simulink subsystem "Compute_Environments"  (R2025b)
settings: Solver=VariableStepAuto  StartTime=0.0  StopTime=10.0  RelTol=1e-3
undefined symbols (not defined in the file): alpha_temp, Cbar, g0, gamma, h_0_2, magnitude, mu0, P_0_1, P_0_2, r_planet_radius, Rair, rho_0_1, rho_0_2, S, T_0_1, T_0_2
settings Model: Creator=Kat  LastModifiedBy=cdriggs

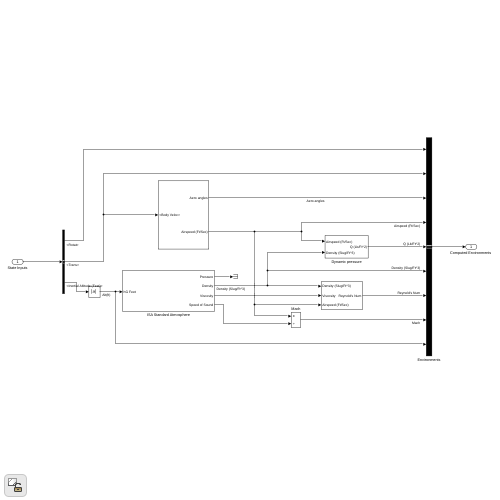
[thumbnail: Simulink's stored preview of the top-level diagram]
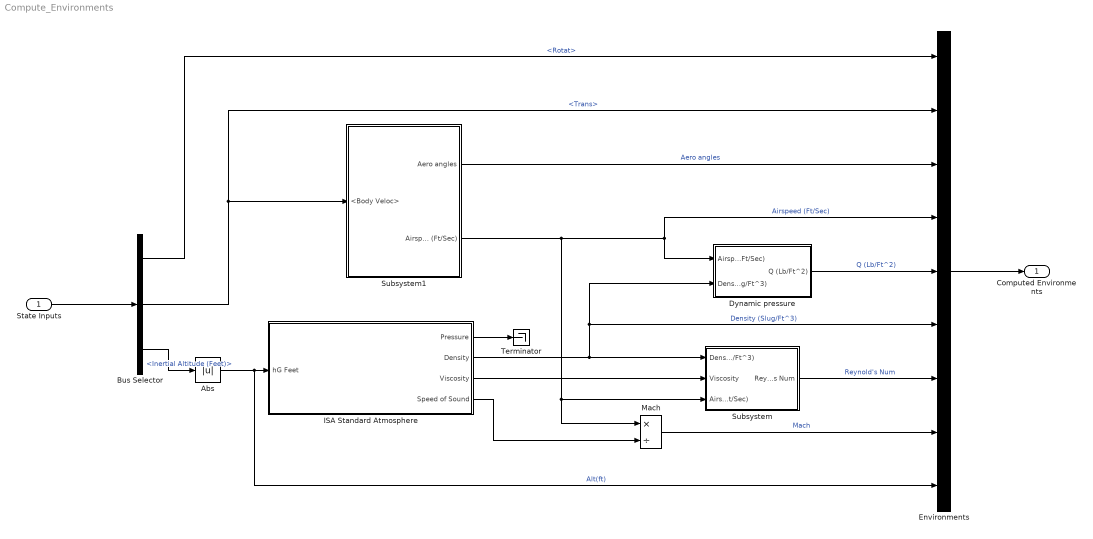
== system Compute_Environments ==
  State Inputs : Inport
  Abs : Abs  SaturateOnIntegerOverflow=off
  Bus Selector : BusSelector  OutputSignals=Rotat,Trans,Trans.Inertial Pos.Inertial Altitude (Feet)
  Dynamic pressure : Subsystem
  Environments : BusCreator  Inputs=9
  ISA Standard Atmosphere : Subsystem
  Mach : Product  Inputs=*/
  Subsystem : Subsystem
  Subsystem1 : Subsystem
  Terminator : Terminator
  "Computed Environments " : Outport
  wires:
  Subsystem1/2(Airspeed (Ft/Sec)) -> Subsystem/3(Airspeed (Ft/Sec)), Mach/1, Dynamic pressure/1(Airspeed (Ft/Sec)), Environments/4  "Airspeed (Ft/Sec)"
  Dynamic pressure/1(Q (Lb/Ft^2)) -> Environments/5  "Q (Lb/Ft^2)"
  Bus Selector/2 -> Subsystem1/1(<Body Veloc>), Environments/2  "<Trans>"
  Subsystem/1(Reynold's Num) -> Environments/7  "Reynold's Num"
  Environments/1 -> "Computed Environments "/1
  Mach/1 -> Environments/8  "Mach"
  State Inputs/1 -> Bus Selector/1
  Bus Selector/1 -> Environments/1  "<Rotat>"
  Subsystem1/1(Aero angles) -> Environments/3  "Aero angles"
  ISA Standard Atmosphere/3(Viscosity) -> Subsystem/2(Viscosity)
  ISA Standard Atmosphere/4(Speed of Sound) -> Mach/2
  ISA Standard Atmosphere/1(Pressure) -> Terminator/1
  ISA Standard Atmosphere/2(Density) -> Subsystem/1(Density (Slug/Ft^3)), Environments/6, Dynamic pressure/2(Density (Slug/Ft^3))  "Density (Slug/Ft^3)"
  Bus Selector/3 -> Abs/1  "<Inertial Altitude (Feet)>"
  Abs/1 -> ISA Standard Atmosphere/1(hG Feet), Environments/9  "Alt(ft)"

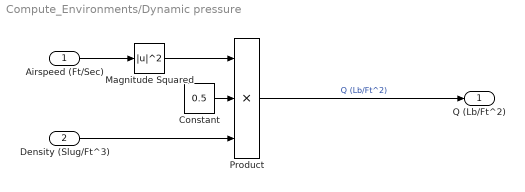
== system Compute_Environments/Dynamic pressure ==
  Airspeed (Ft/Sec) : Inport
  Density (Slug/Ft^3) : Inport  Port=2
  Constant : Constant  Value=0.5
  Magnitude Squared : Math  Operator=magnitude^2
  Product : Product  Inputs=3
  Q (Lb/Ft^2) : Outport
  wires:
  Constant/1 -> Product/2
  Magnitude Squared/1 -> Product/1
  Density (Slug/Ft^3)/1 -> Product/3
  Airspeed (Ft/Sec)/1 -> Magnitude Squared/1
  Product/1 -> Q (Lb/Ft^2)/1  "Q (Lb/Ft^2)"

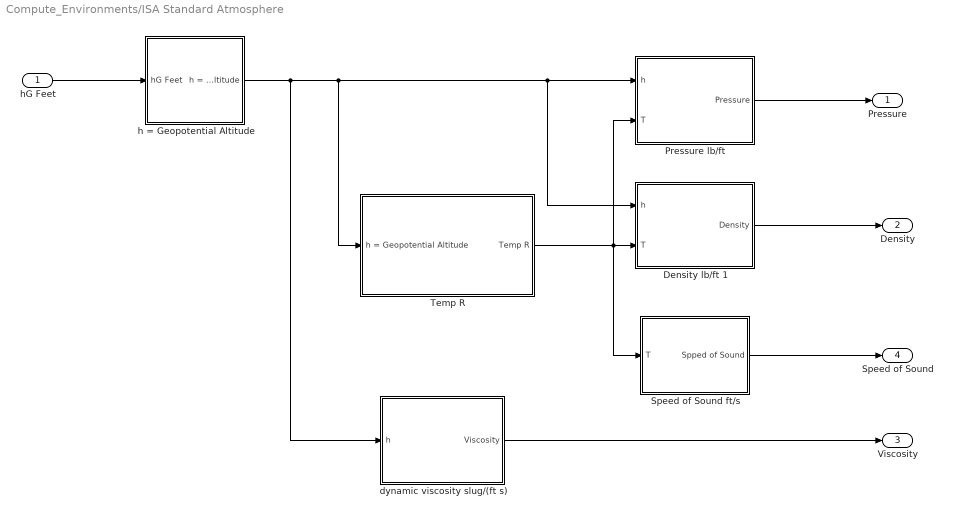
== system Compute_Environments/ISA Standard Atmosphere ==
  hG Feet : Inport
  Density lb/ft 1 : Subsystem
  "Pressure lb/ft " : Subsystem
  Speed of Sound ft/s : Subsystem
  Temp R : Subsystem
  dynamic viscosity slug/(ft s) : Subsystem
  h = Geopotential Altitude : Subsystem
  Pressure : Outport
  Density : Outport  Port=2
  Viscosity : Outport  Port=3
  Speed of Sound : Outport  Port=4
  wires:
  hG Feet/1 -> h = Geopotential Altitude/1(hG Feet)
  "Pressure lb/ft "/1(Pressure) -> Pressure/1
  Temp R/1(Temp R) -> Speed of Sound ft/s/1(T), Density lb/ft 1/2(T), "Pressure lb/ft "/2(T)
  Density lb/ft 1/1(Density) -> Density/1
  Speed of Sound ft/s/1(Spped of Sound) -> Speed of Sound/1
  dynamic viscosity slug/(ft s)/1(Viscosity) -> Viscosity/1
  h = Geopotential Altitude/1(h = Geopotential Altitude) -> "Pressure lb/ft "/1(h), Density lb/ft 1/1(h), Temp R/1(h = Geopotential Altitude), dynamic viscosity slug/(ft s)/1(h)

== system Compute_Environments/Subsystem ==
  Density (Slug/Ft^3) : Inport
  Viscosity : Inport  Port=2
  Airspeed (Ft/Sec) : Inport  Port=3
  Constant1 : Constant  Value=Cbar
  mult : Product  Inputs=***/
  Reynold's Num : Outport
  wires:
  Constant1/1 -> mult/3
  mult/1 -> Reynold's Num/1  "Reynold's Num"
  Airspeed (Ft/Sec)/1 -> mult/2
  Viscosity/1 -> mult/4
  Density (Slug/Ft^3)/1 -> mult/1

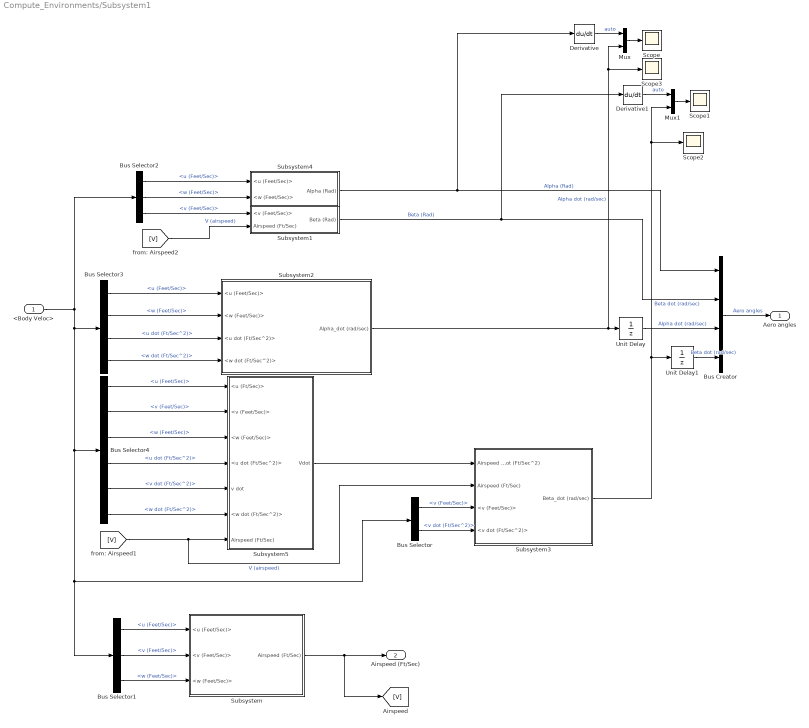
== system Compute_Environments/Subsystem1 ==
  <Body Veloc> : Inport
  Bus Creator : BusCreator  Inputs=4
  Bus Selector : BusSelector  OutputSignals=Body Veloc.v (Feet/Sec),Lin Accels.v dot (Ft/Sec^2)
  Bus Selector1 : BusSelector  OutputSignals=Body Veloc.u (Feet/Sec),Body Veloc.v (Feet/Sec),Body Veloc.w (Feet/Sec)
  Bus Selector2 : BusSelector  OutputSignals=Body Veloc.u (Feet/Sec),Body Veloc.w (Feet/Sec),Body Veloc.v (Feet/Sec)
  Bus Selector3 : BusSelector  OutputSignals=Body Veloc.u (Feet/Sec),Body Veloc.w (Feet/Sec),Lin Accels.u dot (Ft/Sec^2),Lin Accels.w dot (Ft/Sec^2)
  Bus Selector4 : BusSelector  OutputSignals=Body Veloc.u (Feet/Sec),Body Veloc.v (Feet/Sec),Body Veloc.w (Feet/Sec),Lin Accels.u dot (Ft/Sec^2),Lin Accels.v dot (Ft/Sec^2),Lin Accels.w dot (Ft/Sec^2)
  Derivative : Derivative
  Derivative1 : Derivative
  Mux : Mux  Inputs=2
  Mux1 : Mux  Inputs=2
  Scope{,1..3} (4 alike) : Scope
      Scope settings: ActiveDisplayYMinimum=-0.0012525958255160388  ActiveDisplayYMaximum=0.0018610833356130711  DataLoggingVariableName=ScopeData12
      Scope1 settings: ActiveDisplayYMinimum=-5.72624977757219E-20  ActiveDisplayYMaximum=5.5763683770522856E-20  DataLoggingVariableName=ScopeData13
      Scope2 settings: ActiveDisplayYMinimum=-1.0950671202531648  ActiveDisplayYMaximum=1.1099328797468351  DataLoggingVariableName=ScopeData14
      Scope3 settings: ActiveDisplayYMinimum=-0.0012525958255160388  ActiveDisplayYMaximum=0.0018610833356130711  DataLoggingVariableName=ScopeData15
  Subsystem : Subsystem
  Subsystem1 : Subsystem
  Subsystem2 : Subsystem
  Subsystem3 : Subsystem
  Subsystem4 : Subsystem
  Subsystem5 : Subsystem
  Unit Delay : UnitDelay  SampleTime=-1  HasFrameUpgradeWarning=on
  Unit Delay1 : UnitDelay  SampleTime=-1  HasFrameUpgradeWarning=on
  Aero angles : Outport
  Airspeed (Ft/Sec) : Outport  Port=2
  wires:
  Unit Delay1/1 -> Bus Creator/4  "Beta dot (rad/sec)"
  Unit Delay/1 -> Bus Creator/3  "Alpha dot (rad/sec)"
  Subsystem2/1(Alpha_dot (rad/sec)) -> Unit Delay/1, Mux/2, Scope3/1  "Alpha dot (rad/sec)"
  Derivative1/1 -> Mux1/1  "auto"
  Mux1/1 -> Scope1/1
  Derivative/1 -> Mux/1  "auto"
  Mux/1 -> Scope/1
  Bus Creator/1 -> Aero angles/1  "Aero angles"
  Bus Selector2/3 -> Subsystem1/1(<v (Feet/Sec)>)  "<v (Feet/Sec)>"
  [V] -> Subsystem1/2(Airspeed (Ft/Sec))  "V (airspeed)"
  Bus Selector/2 -> Subsystem3/4(<v dot (Ft/Sec^2)>)  "<v dot (Ft/Sec^2)>"
  Bus Selector/1 -> Subsystem3/3(<v (Feet/Sec)>)  "<v (Feet/Sec)>"
  Subsystem5/1(Vdot) -> Subsystem3/1(Airspeed dot (Ft/Sec^2))
  [V] -> Subsystem5/7(Airspeed (Ft/Sec)), Subsystem3/2(Airspeed (Ft/Sec))  "V (airspeed)"
  Bus Selector4/6 -> Subsystem5/6(<w dot (Ft/Sec^2)>)  "<w dot (Ft/Sec^2)>"
  Bus Selector4/5 -> Subsystem5/5(v dot)  "<v dot (Ft/Sec^2)>"
  Bus Selector4/4 -> Subsystem5/4(<u dot (Ft/Sec^2)>)  "<u dot (Ft/Sec^2)>"
  Bus Selector4/3 -> Subsystem5/3(<w (Feet/Sec)>)  "<w (Feet/Sec)>"
  Bus Selector4/2 -> Subsystem5/2(<v (Feet/Sec)>)  "<v (Feet/Sec)>"
  Bus Selector4/1 -> Subsystem5/1(<u (Ft/Sec)>)  "<u (Feet/Sec)>"
  Bus Selector3/4 -> Subsystem2/4(<w dot (Ft/Sec^2)>)  "<w dot (Ft/Sec^2)>"
  Bus Selector3/3 -> Subsystem2/3(<u dot (Ft/Sec^2)>)  "<u dot (Ft/Sec^2)>"
  Bus Selector3/2 -> Subsystem2/2(<w (Feet/Sec)>)  "<w (Feet/Sec)>"
  Bus Selector3/1 -> Subsystem2/1(<u (Feet/Sec)>)  "<u (Feet/Sec)>"
  Bus Selector2/2 -> Subsystem4/2(<w (Feet/Sec)>)  "<w (Feet/Sec)>"
  Bus Selector2/1 -> Subsystem4/1(<u (Feet/Sec)>)  "<u (Feet/Sec)>"
  Subsystem4/1(Alpha (Rad)) -> Bus Creator/1, Derivative/1  "Alpha (Rad)"
  Subsystem3/1(Beta_dot (rad/sec)) -> Unit Delay1/1, Mux1/2, Scope2/1  "Beta dot (rad/sec)"
  Subsystem1/1(Beta (Rad)) -> Bus Creator/2, Derivative1/1  "Beta (Rad)"
  Subsystem/1(Airspeed (Ft/Sec)) -> Airspeed (Ft/Sec)/1, [V]
  Bus Selector1/2 -> Subsystem/2(<v (Feet/Sec)>)  "<v (Feet/Sec)>"
  Bus Selector1/1 -> Subsystem/1(<u (Feet/Sec)>)  "<u (Feet/Sec)>"
  Bus Selector1/3 -> Subsystem/3(<w (Feet/Sec)>)  "<w (Feet/Sec)>"
  <Body Veloc>/1 -> Bus Selector2/1, Bus Selector3/1, Bus Selector4/1, Bus Selector/1, Bus Selector1/1

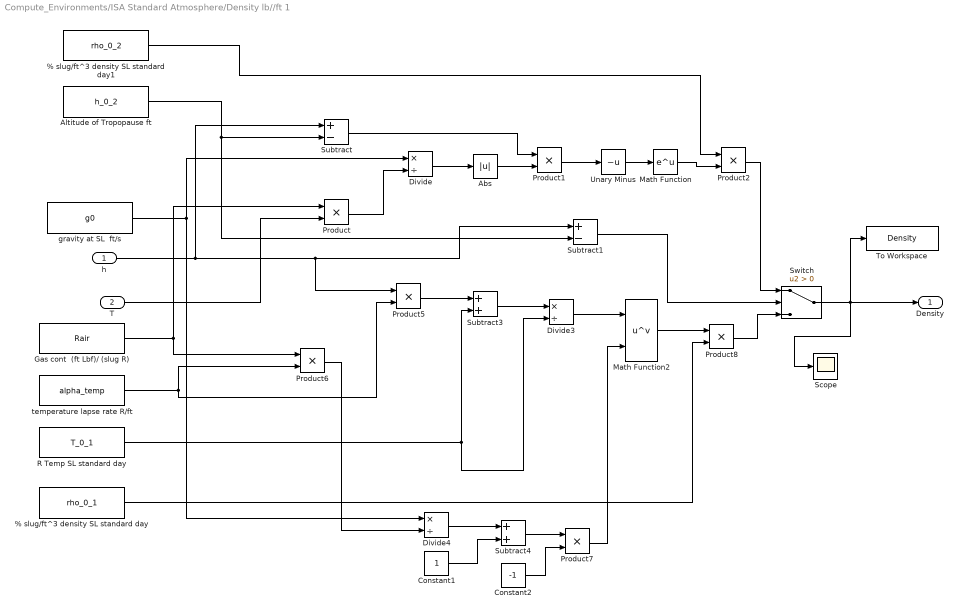
== system Compute_Environments/ISA Standard Atmosphere/Density lb//ft 1 ==
  h : Inport
  T : Inport  Port=2
  " Altitude of Tropopause ft" : Constant  Value=h_0_2
  % slug/ft^3 density SL standard day : Constant  Value=rho_0_1
  % slug/ft^3 density SL standard day1 : Constant  Value=rho_0_2
  Abs : Abs  SaturateOnIntegerOverflow=off
  Constant1 : Constant
  Constant2 : Constant  Value=-1
  Divide : Product  Inputs=*/
  Divide3 : Product  Inputs=*/
  Divide4 : Product  Inputs=*/
  Gas cont  (ft Lbf)/ (slug R) : Constant  Value=Rair
  Math Function : Math
  Math Function2 : Math  Operator=pow
  Product{,1..2,5..8} (7 alike) : Product
  R Temp SL standard day : Constant  Value=T_0_1
  Scope : Scope
      settings: ActiveDisplayYMinimum=0.0006192109618313802  ActiveDisplayYMaximum=0.00079197848153767555  DataLoggingVariableName=ScopeData9
  Subtract : Sum  Inputs=+-
  Subtract1 : Sum  Inputs=+-
  Subtract3 : Sum
  Subtract4 : Sum
  Switch : Switch  Criteria=u2 > Threshold  SaturateOnIntegerOverflow=off  InputSameDT=off
  To Workspace : ToWorkspace  VariableName=Density  SaveFormat=Structure  SampleTime=-1
      settings: MaxDataPoints=1
  Unary Minus : UnaryMinus
  gravity at SL  ft/s : Constant  Value=g0
  temperature lapse rate R/ft : Constant  Value=alpha_temp
  Density : Outport
  wires:
  Gas cont  (ft Lbf)/ (slug R)/1 -> Product/1, Product6/1
  T/1 -> Product/2
  gravity at SL  ft/s/1 -> Divide/1, Divide4/1
  Product/1 -> Divide/2
  Divide/1 -> Abs/1
  Abs/1 -> Product1/2
  Subtract/1 -> Product1/1
  Product1/1 -> Unary Minus/1
  Unary Minus/1 -> Math Function/1
  Math Function/1 -> Product2/2
  % slug/ft^3 density SL standard day1/1 -> Product2/1
  " Altitude of Tropopause ft"/1 -> Subtract1/2, Subtract/2
  Product2/1 -> Switch/1
  Subtract1/1 -> Switch/2
  h/1 -> Subtract/1, Product5/1, Subtract1/1
  Switch/1 -> To Workspace/1, Density/1, Scope/1
  temperature lapse rate R/ft/1 -> Product5/2, Product6/2
  R Temp SL standard day/1 -> Divide3/2, Subtract3/2
  Product5/1 -> Subtract3/1
  Subtract3/1 -> Divide3/1
  Divide3/1 -> Math Function2/1
  Product6/1 -> Divide4/2
  Divide4/1 -> Subtract4/1
  Constant1/1 -> Subtract4/2
  Subtract4/1 -> Product7/1
  Constant2/1 -> Product7/2
  Product7/1 -> Math Function2/2
  Product8/1 -> Switch/3
  Math Function2/1 -> Product8/1
  % slug/ft^3 density SL standard day/1 -> Product8/2

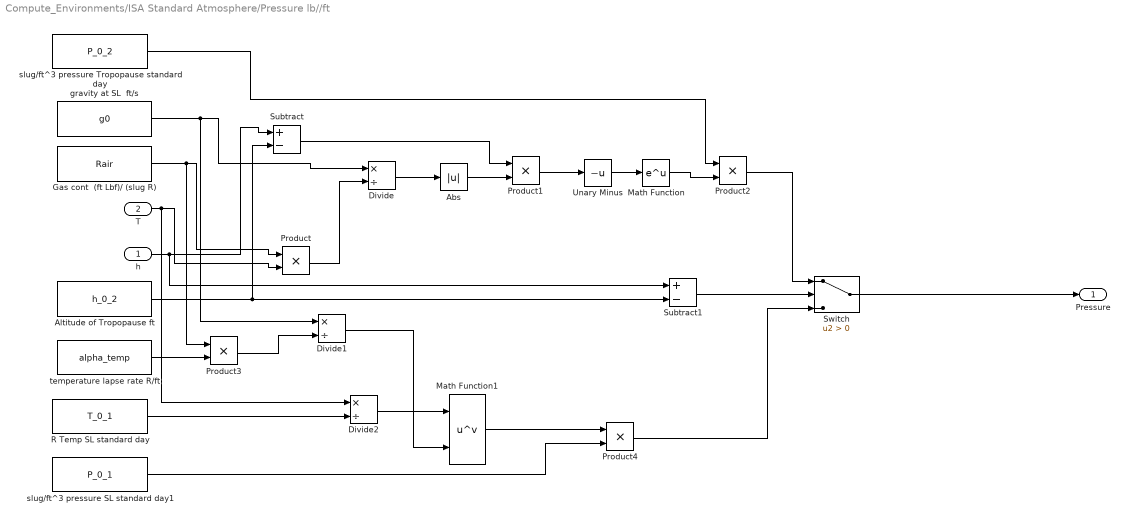
== system Compute_Environments/ISA Standard Atmosphere/Pressure lb//ft  ==
  h : Inport
  T : Inport  Port=2
  " Altitude of Tropopause ft" : Constant  Value=h_0_2
  " slug/ft^3 pressure SL standard day1" : Constant  Value=P_0_1
  " slug/ft^3 pressure Tropopause standard day" : Constant  Value=P_0_2
  Abs : Abs  SaturateOnIntegerOverflow=off
  Divide : Product  Inputs=*/
  Divide1 : Product  Inputs=*/
  Divide2 : Product  Inputs=*/
  Gas cont  (ft Lbf)/ (slug R) : Constant  Value=Rair
  Math Function : Math
  Math Function1 : Math  Operator=pow
  Product{,1..4} (5 alike) : Product
  R Temp SL standard day : Constant  Value=T_0_1
  Subtract : Sum  Inputs=+-
  Subtract1 : Sum  Inputs=+-
  Switch : Switch  Criteria=u2 > Threshold  SaturateOnIntegerOverflow=off  InputSameDT=off
  Unary Minus : UnaryMinus
  gravity at SL  ft/s : Constant  Value=g0
  temperature lapse rate R/ft : Constant  Value=alpha_temp
  Pressure : Outport
  wires:
  Gas cont  (ft Lbf)/ (slug R)/1 -> Product3/1, Product/1
  T/1 -> Divide2/1, Product/2
  gravity at SL  ft/s/1 -> Divide1/1, Divide/1
  Product/1 -> Divide/2
  Divide/1 -> Abs/1
  Abs/1 -> Product1/2
  Subtract/1 -> Product1/1
  Product1/1 -> Unary Minus/1
  Unary Minus/1 -> Math Function/1
  Math Function/1 -> Product2/2
  " slug/ft^3 pressure Tropopause standard day"/1 -> Product2/1
  temperature lapse rate R/ft/1 -> Product3/2
  Product3/1 -> Divide1/2
  R Temp SL standard day/1 -> Divide2/2
  Divide2/1 -> Math Function1/1
  Divide1/1 -> Math Function1/2
  " slug/ft^3 pressure SL standard day1"/1 -> Product4/2
  Math Function1/1 -> Product4/1
  Product4/1 -> Switch/3
  h/1 -> Subtract1/1, Subtract/1
  Product2/1 -> Switch/1
  Subtract1/1 -> Switch/2
  Switch/1 -> Pressure/1
  " Altitude of Tropopause ft"/1 -> Subtract1/2, Subtract/2

== system Compute_Environments/ISA Standard Atmosphere/Speed of Sound ft//s ==
  T : Inport
  Gas cont  (ft Lbf)/ (slug R) : Constant  Value=Rair
  Product : Product  Inputs=3
  Sqrt : Sqrt
  gamma = 1.4; : Constant  Value=gamma
  Spped of Sound : Outport
  wires:
  Gas cont  (ft Lbf)/ (slug R)/1 -> Product/1
  T/1 -> Product/2
  gamma = 1.4;/1 -> Product/3
  Product/1 -> Sqrt/1
  Sqrt/1 -> Spped of Sound/1

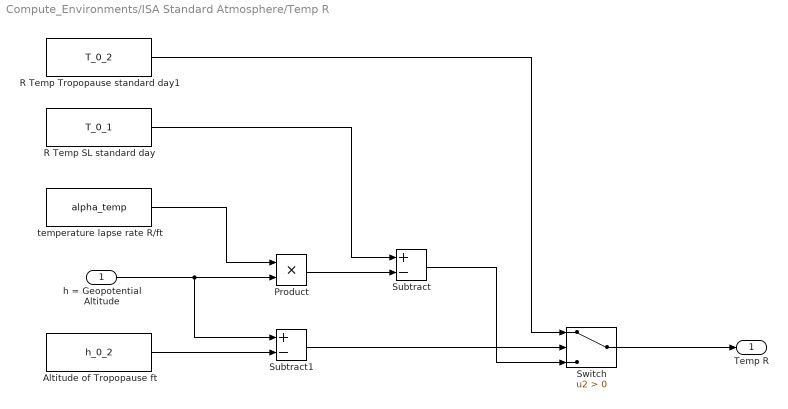
== system Compute_Environments/ISA Standard Atmosphere/Temp R ==
  h = Geopotential Altitude : Inport
  " Altitude of Tropopause ft" : Constant  Value=h_0_2
  Product : Product
  R Temp SL standard day : Constant  Value=T_0_1
  R Temp Tropopause standard day1 : Constant  Value=T_0_2
  Subtract : Sum  Inputs=+-
  Subtract1 : Sum  Inputs=+-
  Switch : Switch  Criteria=u2 > Threshold  SaturateOnIntegerOverflow=off  InputSameDT=off
  temperature lapse rate R/ft : Constant  Value=alpha_temp
  Temp R : Outport
  wires:
  Subtract/1 -> Switch/3
  Product/1 -> Subtract/2
  R Temp SL standard day/1 -> Subtract/1
  R Temp Tropopause standard day1/1 -> Switch/1
  temperature lapse rate R/ft/1 -> Product/1
  Switch/1 -> Temp R/1
  " Altitude of Tropopause ft"/1 -> Subtract1/2
  Subtract1/1 -> Switch/2
  h = Geopotential Altitude/1 -> Subtract1/1, Product/2

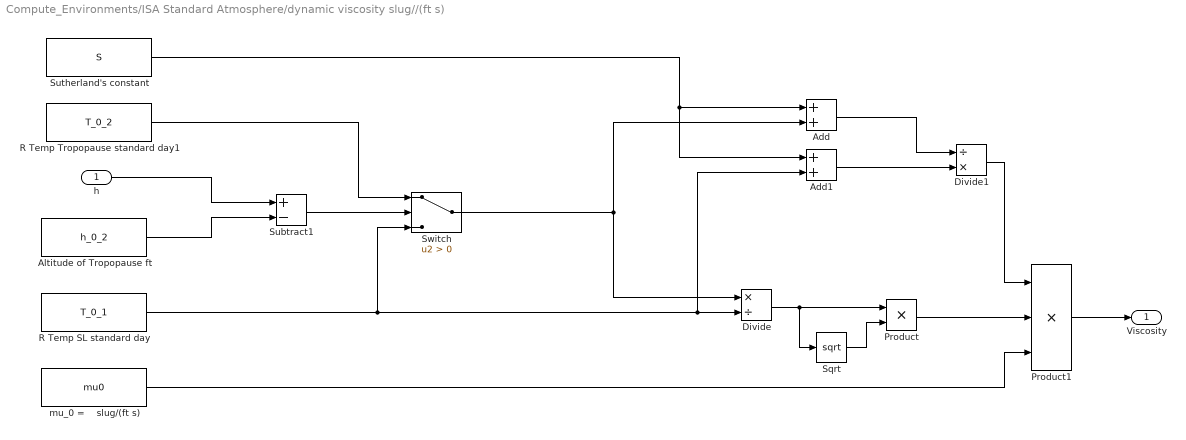
== system Compute_Environments/ISA Standard Atmosphere/dynamic viscosity slug//(ft s) ==
  h : Inport
  " Altitude of Tropopause ft" : Constant  Value=h_0_2
  Add : Sum
  Add1 : Sum
  Divide : Product  Inputs=*/
  Divide1 : Product  Inputs=/*
  Product : Product
  Product1 : Product  Inputs=3
  R Temp SL standard day : Constant  Value=T_0_1
  R Temp Tropopause standard day1 : Constant  Value=T_0_2
  Sqrt : Sqrt
  Subtract1 : Sum  Inputs=+-
  "Sutherland's constant " : Constant  Value=S
  Switch : Switch  Criteria=u2 > Threshold  SaturateOnIntegerOverflow=off  InputSameDT=off
  "mu_0 =    slug/(ft s) " : Constant  Value=mu0
  Viscosity : Outport
  wires:
  Switch/1 -> Add/2, Divide/1
  R Temp SL standard day/1 -> Switch/3, Add1/2, Divide/2
  Divide/1 -> Product/1, Sqrt/1
  Sqrt/1 -> Product/2
  "Sutherland's constant "/1 -> Add1/1, Add/1
  Add1/1 -> Divide1/2
  Add/1 -> Divide1/1
  Product/1 -> Product1/2
  Product1/1 -> Viscosity/1
  Subtract1/1 -> Switch/2
  h/1 -> Subtract1/1
  " Altitude of Tropopause ft"/1 -> Subtract1/2
  R Temp Tropopause standard day1/1 -> Switch/1
  "mu_0 =    slug/(ft s) "/1 -> Product1/3
  Divide1/1 -> Product1/1

== system Compute_Environments/ISA Standard Atmosphere/h = Geopotential Altitude ==
  hG Feet : Inport
  Add : Sum
  Divide : Product  Inputs=*/
  Product : Product
  r = radius of E ft1 : Constant  Value=r_planet_radius
  h = Geopotential Altitude : Outport
  wires:
  r = radius of E ft1/1 -> Add/2, Divide/1
  Add/1 -> Divide/2
  Divide/1 -> Product/2
  hG Feet/1 -> Product/1, Add/1
  Product/1 -> h = Geopotential Altitude/1

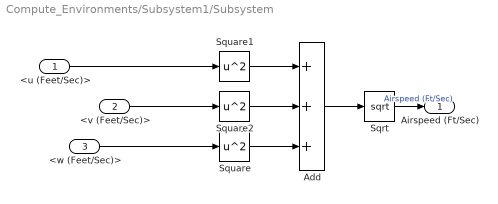
== system Compute_Environments/Subsystem1/Subsystem ==
  <u (Feet/Sec)> : Inport
  <v (Feet/Sec)> : Inport  Port=2
  <w (Feet/Sec)> : Inport  Port=3
  Add : Sum  Inputs=+++
  Sqrt : Sqrt
  Square : Math  Operator=square
  Square1 : Math  Operator=square
  Square2 : Math  Operator=square
  Airspeed (Ft/Sec) : Outport
  wires:
  Sqrt/1 -> Airspeed (Ft/Sec)/1  "Airspeed (Ft/Sec)"
  Square/1 -> Add/3
  <v (Feet/Sec)>/1 -> Square2/1
  <w (Feet/Sec)>/1 -> Square/1
  <u (Feet/Sec)>/1 -> Square1/1
  Square2/1 -> Add/2
  Add/1 -> Sqrt/1
  Square1/1 -> Add/1

== system Compute_Environments/Subsystem1/Subsystem1 ==
  <v (Feet/Sec)> : Inport
  Airspeed (Ft/Sec) : Inport  Port=2
  Asin : Trigonometry  Operator=asin
  Divide : Product  Inputs=*/
  Beta (Rad) : Outport
  wires:
  Airspeed (Ft/Sec)/1 -> Divide/2
  <v (Feet/Sec)>/1 -> Divide/1
  Divide/1 -> Asin/1
  Asin/1 -> Beta (Rad)/1  "Beta (Rad)"

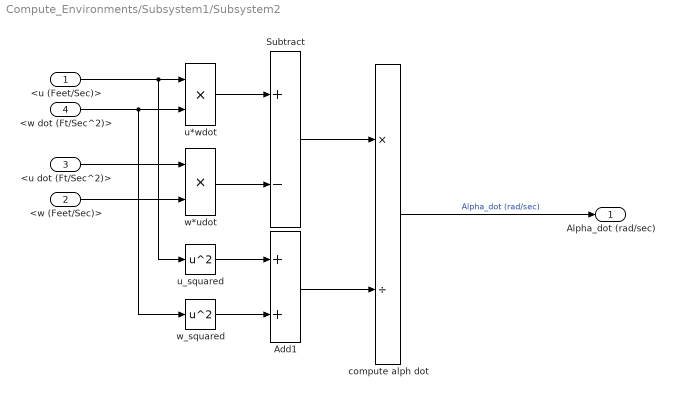
== system Compute_Environments/Subsystem1/Subsystem2 ==
  <u (Feet/Sec)> : Inport
  <w (Feet/Sec)> : Inport  Port=2
  <u dot (Ft/Sec^2)> : Inport  Port=3
  <w dot (Ft/Sec^2)> : Inport  Port=4
  Add1 : Sum
  Subtract : Sum  Inputs=+-
  compute alph dot : Product  Inputs=*/
  u*wdot : Product
  u_squared : Math  Operator=square
  w*udot : Product
  w_squared : Math  Operator=square
  Alpha_dot (rad/sec) : Outport
  wires:
  u_squared/1 -> Add1/1
  <u (Feet/Sec)>/1 -> u*wdot/1, u_squared/1
  compute alph dot/1 -> Alpha_dot (rad/sec)/1  "Alpha_dot (rad/sec)"
  <w (Feet/Sec)>/1 -> w*udot/2
  u*wdot/1 -> Subtract/1
  <u dot (Ft/Sec^2)>/1 -> w*udot/1
  Subtract/1 -> compute alph dot/1
  Add1/1 -> compute alph dot/2
  w_squared/1 -> Add1/2
  <w dot (Ft/Sec^2)>/1 -> u*wdot/2, w_squared/1
  w*udot/1 -> Subtract/2

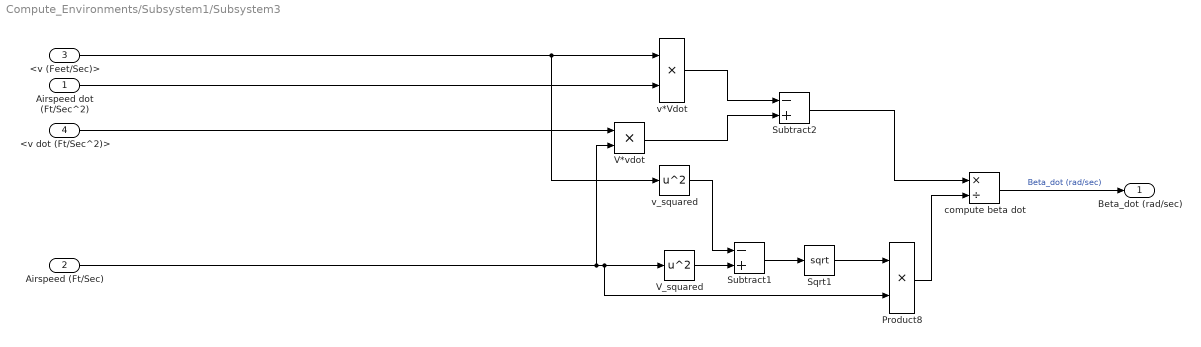
== system Compute_Environments/Subsystem1/Subsystem3 ==
  Airspeed dot (Ft/Sec^2) : Inport
  Airspeed (Ft/Sec) : Inport  Port=2
  <v (Feet/Sec)> : Inport  Port=3
  <v dot (Ft/Sec^2)> : Inport  Port=4
  Product8 : Product
  Sqrt1 : Sqrt
  Subtract1 : Sum  Inputs=-+
  Subtract2 : Sum  Inputs=-+
  V*vdot : Product
  V_squared : Math  Operator=square
  compute beta dot : Product  Inputs=*/
  v*Vdot : Product
  v_squared : Math  Operator=square
  Beta_dot (rad/sec) : Outport
  wires:
  Airspeed dot (Ft/Sec^2)/1 -> v*Vdot/2
  <v (Feet/Sec)>/1 -> v*Vdot/1, v_squared/1
  Subtract2/1 -> compute beta dot/1
  V*vdot/1 -> Subtract2/2
  Sqrt1/1 -> Product8/1
  Product8/1 -> compute beta dot/2
  <v dot (Ft/Sec^2)>/1 -> V*vdot/1
  compute beta dot/1 -> Beta_dot (rad/sec)/1  "Beta_dot (rad/sec)"
  Airspeed (Ft/Sec)/1 -> V_squared/1, Product8/2, V*vdot/2
  V_squared/1 -> Subtract1/2
  v*Vdot/1 -> Subtract2/1
  v_squared/1 -> Subtract1/1
  Subtract1/1 -> Sqrt1/1

== system Compute_Environments/Subsystem1/Subsystem4 ==
  <u (Feet/Sec)> : Inport
  <w (Feet/Sec)> : Inport  Port=2
  Atan2 : Trigonometry  Operator=atan2
  Alpha (Rad) : Outport
  wires:
  Atan2/1 -> Alpha (Rad)/1  "Alpha (Rad)"
  <u (Feet/Sec)>/1 -> Atan2/2
  <w (Feet/Sec)>/1 -> Atan2/1

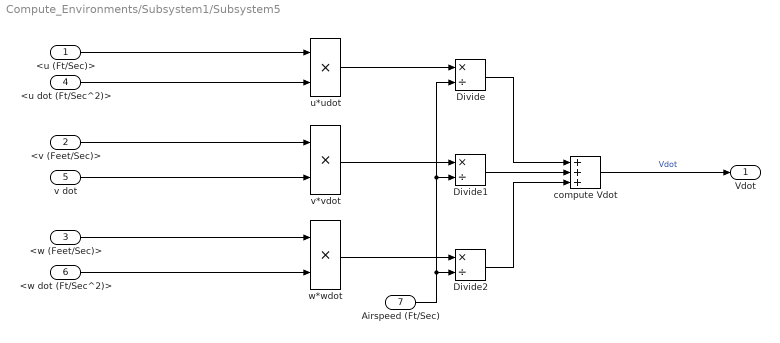
== system Compute_Environments/Subsystem1/Subsystem5 ==
  <u (Ft/Sec)> : Inport
  <v (Feet/Sec)> : Inport  Port=2
  <w (Feet/Sec)> : Inport  Port=3
  <u dot (Ft/Sec^2)> : Inport  Port=4
  v dot : Inport  Port=5
  <w dot (Ft/Sec^2)> : Inport  Port=6
  Airspeed (Ft/Sec) : Inport  Port=7
  Divide : Product  Inputs=*/
  Divide1 : Product  Inputs=*/
  Divide2 : Product  Inputs=*/
  compute Vdot : Sum  Inputs=+++
  u*udot : Product
  v*vdot : Product
  w*wdot : Product
  Vdot : Outport
  wires:
  u*udot/1 -> Divide/1
  w*wdot/1 -> Divide2/1
  <v (Feet/Sec)>/1 -> v*vdot/1
  <u dot (Ft/Sec^2)>/1 -> u*udot/2
  Divide2/1 -> compute Vdot/3
  v dot/1 -> v*vdot/2
  compute Vdot/1 -> Vdot/1  "Vdot"
  Divide1/1 -> compute Vdot/2
  v*vdot/1 -> Divide1/1
  <w (Feet/Sec)>/1 -> w*wdot/1
  <u (Ft/Sec)>/1 -> u*udot/1
  <w dot (Ft/Sec^2)>/1 -> w*wdot/2
  Airspeed (Ft/Sec)/1 -> Divide2/2, Divide1/2, Divide/2
  Divide/1 -> compute Vdot/1
